simulink model "satcom_4axis_inverse_dinamik"  (R2024b)
settings: Solver=FixedStepDiscrete  StartTime=0.0  StopTime=75.5445  FixedStep=0.0050003  RelTol=1e-3
settings Model: Creator=user  LastModifiedBy=user
settings DataIOCC: ExternalInput=in_qdot_az, in_qddot_az, in_zero, in_zero, in_zero, in_zero, in_zero, in_zero  LoadExternalInput=on

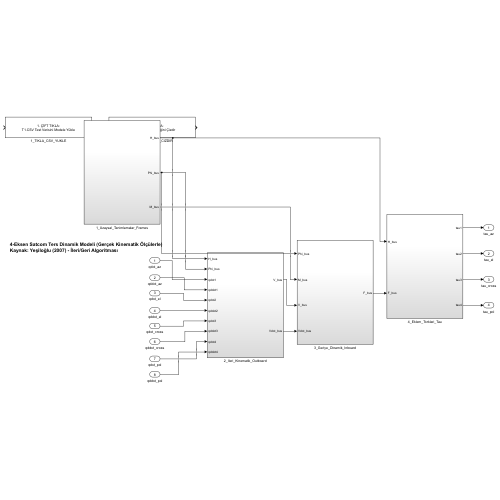
[thumbnail: Simulink's stored preview of the top-level diagram]
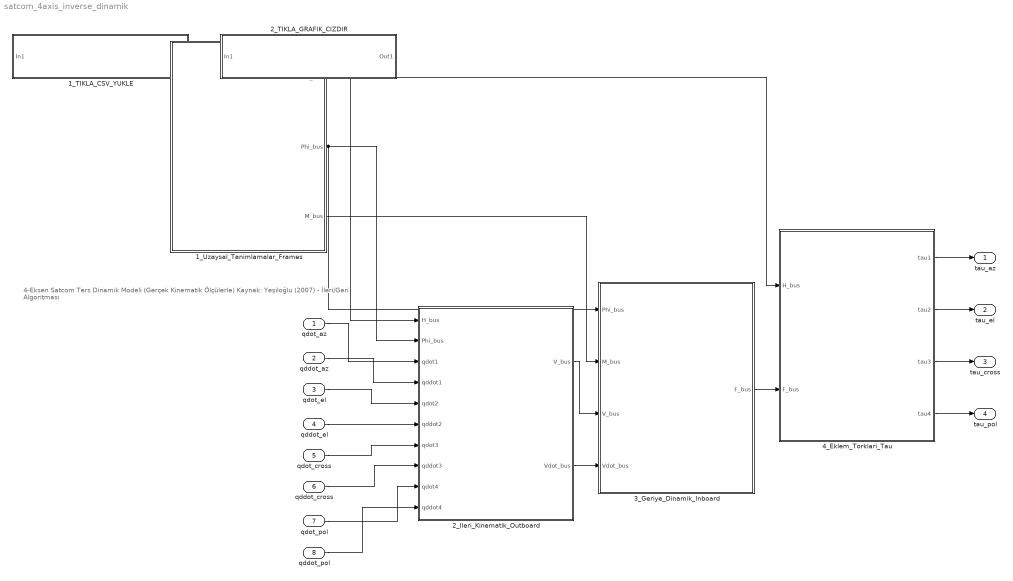
== system satcom_4axis_inverse_dinamik ==
  note: 4-Eksen Satcom Ters Dinamik Modeli (Gerçek Kinematik Ölçülerle)
      | Kaynak: Yeşiloğlu (2007) - İleri/Geri Algoritması
  qdot_az : Inport
  qddot_az : Inport  Port=2
  qdot_el : Inport  Port=3
  qddot_el : Inport  Port=4
  qdot_cross : Inport  Port=5
  qddot_cross : Inport  Port=6
  qdot_pol : Inport  Port=7
  qddot_pol : Inport  Port=8
  1_TIKLA_CSV_YUKLE : Subsystem
      settings: OpenFcn=try, [f,p]=uigetfile({'*.csv;*.xlsx'}); if f~=0, ham_veri = importdata(fullfile(p,f)); if isstruct(ham_veri), mat = ham_veri.data; else, mat = ham_veri; end, t = mat(:,2); t=t(:); v = mat(:,5); v=v(:); a = mat(:,7); a=a(:); akim = mat(:,9); akim=akim(:); tau_real = akim * 1.41; tau_real=tau_real(:); z = zeros(size(t)); dt_array = diff(t); dt_array(dt_array==0)=1e-6; dt_mean = mean(dt_array); assignin('base','in_qdot_az',timeseries(v,t)); assignin('base','in_qddot_az',timeseries(a,t)); assignin('base','in_zero',timeseries(z,t)); assignin('base','csv_zaman',t); assignin('base','csv_tork',tau_real); set_param(bdroot,'SolverType','Fixed-step'); set_param(bdroot,'Solver','FixedStepDiscrete'); set_param(bdroot,'FixedStep',num2str(dt_mean)); set_param(bdroot,'LoadExternalInput','on'); set_param(bdroot,'ExternalInput','in_qdot_az, in_qddot_az, in_zero, in_zero, in_zero, in_zero, in_zero, in_zero'); set_param(bdroot,'StopTime',num2str(t(end))); msgbox('T1.csv verileri yüklendi! Filtreler ve sınırlandırmalar kaldırıldı.', 'BAŞARILI'); end, catch ME, errordlg(sprintf('HATA:\\n%s', ME.message), 'Sistem Hatası'); end
      mask Display: disp('1. ÇİFT TIKLA:\nT1.CSV Test Verisini Modele Yükle');
  1_Uzaysal_Tanimlamalar_Frames : Subsystem
  2_Ileri_Kinematik_Outboard : Subsystem
  2_TIKLA_GRAFIK_CIZDIR : Subsystem
      settings: OpenFcn=try, simOut = evalin('base', 'out'); tau_raw = double(simOut.yout{1}.Values.Data(:)); t_sim = double(simOut.yout{1}.Values.Time(:)); [t_u, idx] = unique(t_sim); tau_u = tau_raw(idx); zaman = evalin('base', 'csv_zaman'); zaman = zaman(:); tau_real = evalin('base', 'csv_tork'); tau_real = tau_real(:); tau_model = interp1(t_u, tau_u, zaman, 'linear', 'extrap'); tau_model = tau_model(:); figure('Name', 'Dinamik Model vs Gerçek Test', 'NumberTitle', 'off'); plot(zaman, tau_model, 'b', 'LineWidth', 1.5); hold on; plot(zaman, tau_real, 'r--', 'LineWidth', 1.2); title('Azimut Motoru - Tork İhtiyacı (Saf Kinematik Model vs Sürücü)'); xlabel('Zaman (s)'); ylabel('Tork (Nm)'); legend('Model Torku (Gerçek Uzuv Mesafeleri İle)', 'Gerçek Sürücü Torku'); grid on; SonucTablosu = table(zaman, tau_model, tau_real, 'VariableNames', {'Zaman_saniye', 'Model_Uretilen_Tork_Nm', 'Gercek_Sistem_Tork_Referansi'}); writetable(SonucTablosu, 'Model_Tork_Sonuclari.csv'); disp('Doğrulama verileri kaydedildi!'); catch ME, errordlg(sprintf('GRAFİK ÇİZİLEMEDİ!\\n\\nHata:\\n%s', ME.message), 'Sistem Hatası'); end
      mask Display: disp('2. ÇİFT TIKLA:\nSaf Model Tork Grafiğini Çizdir');
  3_Geriye_Dinamik_Inboard : Subsystem
  4_Eklem_Torklari_Tau : Subsystem
  tau_az : Outport
  tau_el : Outport  Port=2
  tau_cross : Outport  Port=3
  tau_pol : Outport  Port=4
  wires:
  qdot_az/1 -> 2_Ileri_Kinematik_Outboard/3(qdot1)
  qddot_az/1 -> 2_Ileri_Kinematik_Outboard/4(qddot1)
  qdot_el/1 -> 2_Ileri_Kinematik_Outboard/5(qdot2)
  qddot_el/1 -> 2_Ileri_Kinematik_Outboard/6(qddot2)
  1_Uzaysal_Tanimlamalar_Frames/1(H_bus) -> 4_Eklem_Torklari_Tau/1(H_bus), 2_Ileri_Kinematik_Outboard/1(H_bus)
  qdot_pol/1 -> 2_Ileri_Kinematik_Outboard/9(qdot4)
  qddot_cross/1 -> 2_Ileri_Kinematik_Outboard/8(qddot3)
  qdot_cross/1 -> 2_Ileri_Kinematik_Outboard/7(qdot3)
  4_Eklem_Torklari_Tau/4(tau4) -> tau_pol/1
  4_Eklem_Torklari_Tau/2(tau2) -> tau_el/1
  1_Uzaysal_Tanimlamalar_Frames/2(Phi_bus) -> 3_Geriye_Dinamik_Inboard/1(Phi_bus), 2_Ileri_Kinematik_Outboard/2(Phi_bus)
  1_Uzaysal_Tanimlamalar_Frames/3(M_bus) -> 3_Geriye_Dinamik_Inboard/2(M_bus)
  qddot_pol/1 -> 2_Ileri_Kinematik_Outboard/10(qddot4)
  2_Ileri_Kinematik_Outboard/1(V_bus) -> 3_Geriye_Dinamik_Inboard/3(V_bus)
  2_Ileri_Kinematik_Outboard/2(Vdot_bus) -> 3_Geriye_Dinamik_Inboard/4(Vdot_bus)
  3_Geriye_Dinamik_Inboard/1(F_bus) -> 4_Eklem_Torklari_Tau/2(F_bus)
  4_Eklem_Torklari_Tau/3(tau3) -> tau_cross/1
  4_Eklem_Torklari_Tau/1(tau1) -> tau_az/1

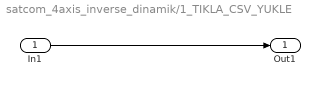
== system satcom_4axis_inverse_dinamik/1_TIKLA_CSV_YUKLE ==
  In1 : Inport
  Out1 : Outport
  wires:
  In1/1 -> Out1/1

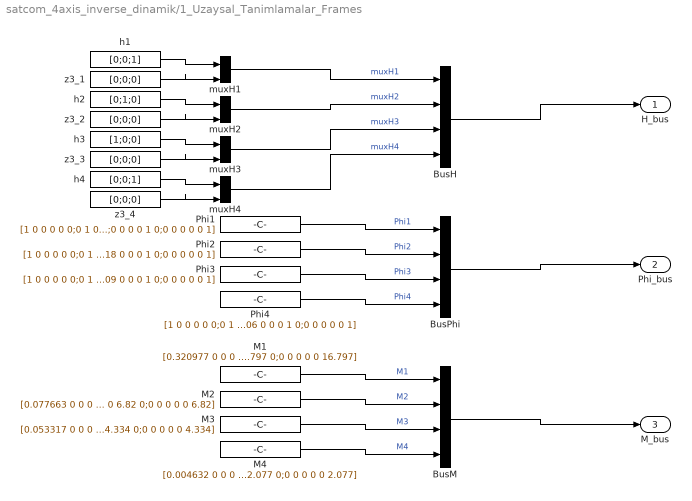
== system satcom_4axis_inverse_dinamik/1_Uzaysal_Tanimlamalar_Frames ==
  BusH : BusCreator  Inputs=4
  BusM : BusCreator  Inputs=4
  BusPhi : BusCreator  Inputs=4
  M1 : Constant  Value=[0.320977 0 0 0 0 0;0 0.320977 0 0 0 0;0 0 0.320977 0 0 0;0 0 0 16.797 0 0;0 0 0 0 16.797 0;0 0 0 0 0 16.797]
  M2 : Constant  Value=[0.077663 0 0 0 0 0;0 0.077663 0 0 0 0;0 0 0.077663 0 0 0;0 0 0 6.82 0 0;0 0 0 0 6.82 0;0 0 0 0 0 6.82]
  M3 : Constant  Value=[0.053317 0 0 0 0 0;0 0.053317 0 0 0 0;0 0 0.053317 0 0 0;0 0 0 4.334 0 0;0 0 0 0 4.334 0;0 0 0 0 0 4.334]
  M4 : Constant  Value=[0.004632 0 0 0 0 0;0 0.004632 0 0 0 0;0 0 0.004632 0 0 0;0 0 0 2.077 0 0;0 0 0 0 2.077 0;0 0 0 0 0 2.077]
  Phi1 : Constant  Value=[1 0 0 0 0 0;0 1 0 0 0 0;0 0 1 0 0 0;0 0 0 1 0 0;0 0 0 0 1 0;0 0 0 0 0 1]
  Phi2 : Constant  Value=[1 0 0 0 0 0;0 1 0 0 0 0;0 0 1 0 0 0;0 0.18 0 1 0 0;-0.18 0 0 0 1 0;0 0 0 0 0 1]
  Phi3 : Constant  Value=[1 0 0 0 0 0;0 1 0 0 0 0;0 0 1 0 0 0;0 0.09 0 1 0 0;-0.09 0 0 0 1 0;0 0 0 0 0 1]
  Phi4 : Constant  Value=[1 0 0 0 0 0;0 1 0 0 0 0;0 0 1 0 0 0;0 0.06 0 1 0 0;-0.06 0 0 0 1 0;0 0 0 0 0 1]
  h1 : Constant  Value=[0;0;1]
  h2 : Constant  Value=[0;1;0]
  h3 : Constant  Value=[1;0;0]
  h4 : Constant  Value=[0;0;1]
  muxH{1..4} (4 alike) : Mux  Inputs=2
  z3_{1..4} (4 alike) : Constant  Value=[0;0;0]
  H_bus : Outport
  Phi_bus : Outport  Port=2
  M_bus : Outport  Port=3
  wires:
  h1/1 -> muxH1/1
  z3_1/1 -> muxH1/2
  muxH1/1 -> BusH/1  "muxH1"
  h2/1 -> muxH2/1
  z3_2/1 -> muxH2/2
  muxH2/1 -> BusH/2  "muxH2"
  h3/1 -> muxH3/1
  z3_3/1 -> muxH3/2
  muxH3/1 -> BusH/3  "muxH3"
  h4/1 -> muxH4/1
  z3_4/1 -> muxH4/2
  muxH4/1 -> BusH/4  "muxH4"
  BusH/1 -> H_bus/1
  Phi1/1 -> BusPhi/1  "Phi1"
  Phi2/1 -> BusPhi/2  "Phi2"
  Phi3/1 -> BusPhi/3  "Phi3"
  Phi4/1 -> BusPhi/4  "Phi4"
  BusPhi/1 -> Phi_bus/1
  M1/1 -> BusM/1  "M1"
  M2/1 -> BusM/2  "M2"
  M3/1 -> BusM/3  "M3"
  M4/1 -> BusM/4  "M4"
  BusM/1 -> M_bus/1

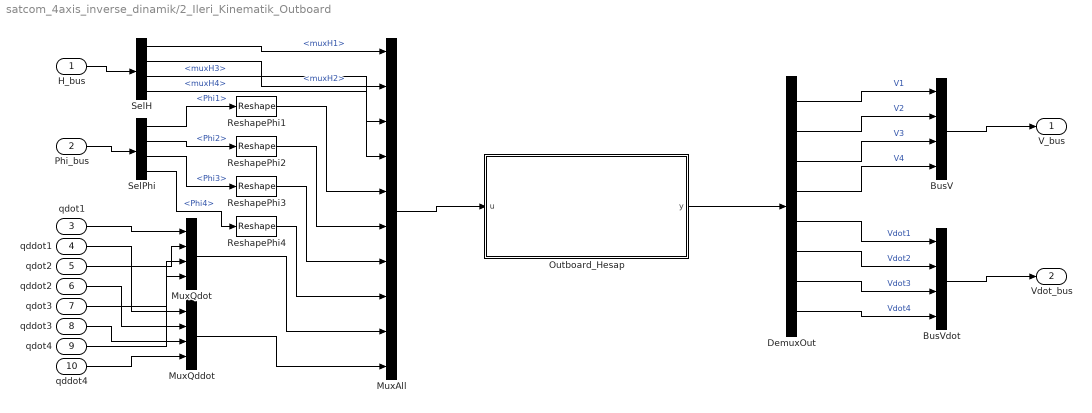
== system satcom_4axis_inverse_dinamik/2_Ileri_Kinematik_Outboard ==
  H_bus : Inport
  Phi_bus : Inport  Port=2
  qdot1 : Inport  Port=3
  qddot1 : Inport  Port=4
  qdot2 : Inport  Port=5
  qddot2 : Inport  Port=6
  qdot3 : Inport  Port=7
  qddot3 : Inport  Port=8
  qdot4 : Inport  Port=9
  qddot4 : Inport  Port=10
  BusV : BusCreator  Inputs=4
  BusVdot : BusCreator  Inputs=4
  DemuxOut : Demux  Outputs=[6 6 6 6 6 6 6 6]
  MuxAll : Mux  Inputs=10
  MuxQddot : Mux
  MuxQdot : Mux
  Outboard_Hesap : MATLAB Function  TreatAsAtomicUnit=on
  ReshapePhi{1..4} (4 alike) : Reshape
  SelH : BusSelector  OutputSignals=muxH1,muxH2,muxH3,muxH4
  SelPhi : BusSelector  OutputSignals=Phi1,Phi2,Phi3,Phi4
  V_bus : Outport
  Vdot_bus : Outport  Port=2
  wires:
  H_bus/1 -> SelH/1
  Phi_bus/1 -> SelPhi/1
  qdot1/1 -> MuxQdot/1
  qddot1/1 -> MuxQddot/1
  qdot2/1 -> MuxQdot/2
  qddot2/1 -> MuxQddot/2
  qdot3/1 -> MuxQdot/3
  qddot3/1 -> MuxQddot/3
  qdot4/1 -> MuxQdot/4
  qddot4/1 -> MuxQddot/4
  SelH/1 -> MuxAll/1  "<muxH1>"
  SelPhi/1 -> ReshapePhi1/1  "<Phi1>"
  ReshapePhi1/1 -> MuxAll/5
  SelH/2 -> MuxAll/2  "<muxH2>"
  SelPhi/2 -> ReshapePhi2/1  "<Phi2>"
  ReshapePhi2/1 -> MuxAll/6
  SelH/3 -> MuxAll/3  "<muxH3>"
  SelPhi/3 -> ReshapePhi3/1  "<Phi3>"
  ReshapePhi3/1 -> MuxAll/7
  SelH/4 -> MuxAll/4  "<muxH4>"
  SelPhi/4 -> ReshapePhi4/1  "<Phi4>"
  ReshapePhi4/1 -> MuxAll/8
  MuxQdot/1 -> MuxAll/9
  MuxQddot/1 -> MuxAll/10
  MuxAll/1 -> Outboard_Hesap/1(u)
  Outboard_Hesap/1(y) -> DemuxOut/1
  DemuxOut/1 -> BusV/1  "V1"
  DemuxOut/5 -> BusVdot/1  "Vdot1"
  DemuxOut/2 -> BusV/2  "V2"
  DemuxOut/6 -> BusVdot/2  "Vdot2"
  DemuxOut/3 -> BusV/3  "V3"
  DemuxOut/7 -> BusVdot/3  "Vdot3"
  DemuxOut/4 -> BusV/4  "V4"
  DemuxOut/8 -> BusVdot/4  "Vdot4"
  BusV/1 -> V_bus/1
  BusVdot/1 -> Vdot_bus/1

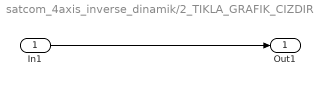
== system satcom_4axis_inverse_dinamik/2_TIKLA_GRAFIK_CIZDIR ==
  In1 : Inport
  Out1 : Outport
  wires:
  In1/1 -> Out1/1

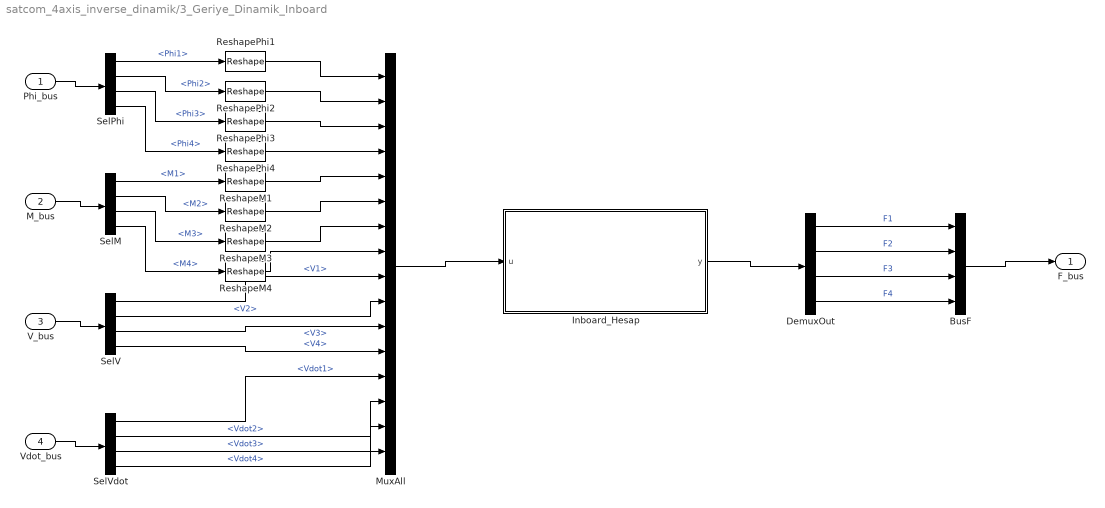
== system satcom_4axis_inverse_dinamik/3_Geriye_Dinamik_Inboard ==
  Phi_bus : Inport
  M_bus : Inport  Port=2
  V_bus : Inport  Port=3
  Vdot_bus : Inport  Port=4
  BusF : BusCreator  Inputs=4
  DemuxOut : Demux  Outputs=[6 6 6 6]
  Inboard_Hesap : MATLAB Function  TreatAsAtomicUnit=on
  MuxAll : Mux  Inputs=16
  ReshapeM{1..4} (4 alike) : Reshape
  ReshapePhi{1..4} (4 alike) : Reshape
  SelM : BusSelector  OutputSignals=M1,M2,M3,M4
  SelPhi : BusSelector  OutputSignals=Phi1,Phi2,Phi3,Phi4
  SelV : BusSelector  OutputSignals=V1,V2,V3,V4
  SelVdot : BusSelector  OutputSignals=Vdot1,Vdot2,Vdot3,Vdot4
  F_bus : Outport
  wires:
  Phi_bus/1 -> SelPhi/1
  M_bus/1 -> SelM/1
  V_bus/1 -> SelV/1
  Vdot_bus/1 -> SelVdot/1
  SelPhi/1 -> ReshapePhi1/1  "<Phi1>"
  ReshapePhi1/1 -> MuxAll/1
  SelM/1 -> ReshapeM1/1  "<M1>"
  ReshapeM1/1 -> MuxAll/5
  SelV/1 -> MuxAll/9  "<V1>"
  SelVdot/1 -> MuxAll/13  "<Vdot1>"
  SelPhi/2 -> ReshapePhi2/1  "<Phi2>"
  ReshapePhi2/1 -> MuxAll/2
  SelM/2 -> ReshapeM2/1  "<M2>"
  ReshapeM2/1 -> MuxAll/6
  SelV/2 -> MuxAll/10  "<V2>"
  SelVdot/2 -> MuxAll/14  "<Vdot2>"
  SelPhi/3 -> ReshapePhi3/1  "<Phi3>"
  ReshapePhi3/1 -> MuxAll/3
  SelM/3 -> ReshapeM3/1  "<M3>"
  ReshapeM3/1 -> MuxAll/7
  SelV/3 -> MuxAll/11  "<V3>"
  SelVdot/3 -> MuxAll/15  "<Vdot3>"
  SelPhi/4 -> ReshapePhi4/1  "<Phi4>"
  ReshapePhi4/1 -> MuxAll/4
  SelM/4 -> ReshapeM4/1  "<M4>"
  ReshapeM4/1 -> MuxAll/8
  SelV/4 -> MuxAll/12  "<V4>"
  SelVdot/4 -> MuxAll/16  "<Vdot4>"
  MuxAll/1 -> Inboard_Hesap/1(u)
  Inboard_Hesap/1(y) -> DemuxOut/1
  DemuxOut/1 -> BusF/1  "F1"
  DemuxOut/2 -> BusF/2  "F2"
  DemuxOut/3 -> BusF/3  "F3"
  DemuxOut/4 -> BusF/4  "F4"
  BusF/1 -> F_bus/1

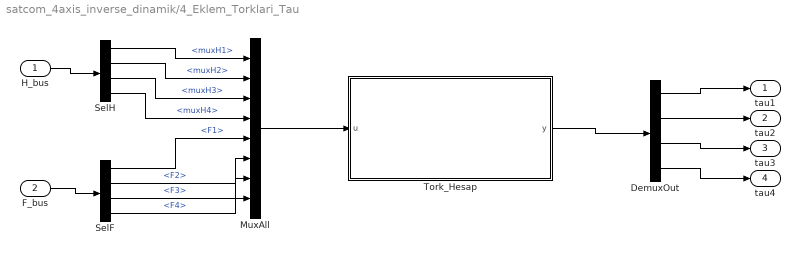
== system satcom_4axis_inverse_dinamik/4_Eklem_Torklari_Tau ==
  H_bus : Inport
  F_bus : Inport  Port=2
  DemuxOut : Demux  Outputs=[1 1 1 1]
  MuxAll : Mux  Inputs=8
  SelF : BusSelector  OutputSignals=F1,F2,F3,F4
  SelH : BusSelector  OutputSignals=muxH1,muxH2,muxH3,muxH4
  Tork_Hesap : MATLAB Function  TreatAsAtomicUnit=on
  tau1 : Outport
  tau2 : Outport  Port=2
  tau3 : Outport  Port=3
  tau4 : Outport  Port=4
  wires:
  H_bus/1 -> SelH/1
  F_bus/1 -> SelF/1
  SelH/1 -> MuxAll/1  "<muxH1>"
  SelF/1 -> MuxAll/5  "<F1>"
  SelH/2 -> MuxAll/2  "<muxH2>"
  SelF/2 -> MuxAll/6  "<F2>"
  SelH/3 -> MuxAll/3  "<muxH3>"
  SelF/3 -> MuxAll/7  "<F3>"
  SelH/4 -> MuxAll/4  "<muxH4>"
  SelF/4 -> MuxAll/8  "<F4>"
  MuxAll/1 -> Tork_Hesap/1(u)
  Tork_Hesap/1(y) -> DemuxOut/1
  DemuxOut/1 -> tau1/1
  DemuxOut/2 -> tau2/1
  DemuxOut/3 -> tau3/1
  DemuxOut/4 -> tau4/1

== matlab function satcom_4axis_inverse_dinamik/2_Ileri_Kinematik_Outboard/Outboard_Hesap ==
  data: u input; y output
function y = fcn(u)
% =========================================================================
% OUTBOARD (ILERI YONLU KINEMATIK) HESAPLAMA BLOGU
% Kaynak: Yesiloglu (2007) - Newton-Euler Ters Dinamik Algoritmasi
% Aciklama: Bu fonksiyonda, kaideden (base) uc is elemanina (end-effector) 
% dogru uzaysal hiz (V) ve uzaysal ivme (Vdot) yayilimini hesapliyorum.
% =========================================================================

H = cell(4,1); Phi = cell(4,1); idx = 1;

% 1. Sinyal Ayiklama: Giris vektorunden H ve Phi matrislerini cekiyoruz
% H: Donme Eksen Vektorleri (Hareket Alt-uzayi matrisleri, 6x1)
for k=1:4, H{k} = u(idx:idx+5); idx = idx + 6; end

% Phi: Uzaysal Donusum (Transfer) Matrisleri (Paralel eksen tasimasi icin, 6x6)
for k=1:4, Phi{k} = reshape(u(idx:idx+35), 6, 6); idx = idx + 36; end

% qdot (Eklem Hizlari) ve qddot (Eklem Ivmeleri)
qdot = u(idx:idx+3); idx = idx + 4; qddot = u(idx:idx+3);

% 2. Baslangic Kosullari: Kaide (Base) sabit oldugu icin hiz ve ivme sifirdir
Vprev = zeros(6,1); Vdotprev = zeros(6,1); V = cell(4,1); Vd = cell(4,1);

% 3. Ileriye Dogru Ozyineleme (Outboard Recursion: 1. eksenden 4. eksene)
for k=1:4
  Vk  = Phi{k}*Vprev + H{k}*qdot(k);
  Vdk = Phi{k}*Vdotprev + H{k}*qddot(k) + crm(Vk)*(H{k}*qdot(k));
  V{k}=Vk; Vd{k}=Vdk; Vprev=Vk; Vdotprev=Vdk;
end

% 4. Cikis Sinyallerini Birlestirme
y = zeros(48,1); idx = 1;
for k=1:4, y(idx:idx+5) = V{k}; idx = idx + 6; end % Uzaysal Hizlar (V1..V4)
for k=1:4, y(idx:idx+5) = Vd{k}; idx = idx + 6; end % Uzaysal Ivmeler (Vdot1..Vdot4)
end

% =========================================================================
% YARDIMCI FONKSIYONLAR
% =========================================================================
function X=crm(V), w=V(1:3); v=V(4:6); X=[skew(w) zeros(3,3); skew(v) skew(w)]; end
function S=skew(a), S=[0 -a(3) a(2); a(3) 0 -a(1); -a(2) a(1) 0]; end

== matlab function satcom_4axis_inverse_dinamik/4_Eklem_Torklari_Tau/Tork_Hesap ==
  data: u input; y output
function y = fcn(u)
H = cell(4,1); F = cell(4,1); idx = 1;
for k=1:4, H{k} = u(idx:idx+5); idx = idx + 6; end
for k=1:4, F{k} = u(idx:idx+5); idx = idx + 6; end
y = zeros(4,1);
for k=1:4
  y(k) = H{k}' * F{k}; 
end
end

== matlab function satcom_4axis_inverse_dinamik/3_Geriye_Dinamik_Inboard/Inboard_Hesap ==
  data: u input; y output
function y = fcn(u)
% =========================================================================
% INBOARD (GERIYE DOGRU DINAMIK) HESAPLAMA BLOGU
% Kaynak: Yesiloglu (2007) - Newton-Euler Ters Dinamik Algoritmasi
% Aciklama: Bu fonksiyonda, en uctaki is elemanindan kaideye dogru 
% geriye isleyerek uzaysal kuvvetlerin yayilimini hesapliyorum.
% =========================================================================

Phi = cell(4,1); I_mat = cell(4,1); V = cell(4,1); Vd = cell(4,1); idx = 1;

% 1. Sinyal Ayiklama: Ileri kinematikten gelen matrisleri ayikliyorum
% Phi: Uzaysal Donusum matrisleri (6x6)
for k=1:4, Phi{k} = reshape(u(idx:idx+35), 6, 6); idx = idx + 36; end

% I_mat: Uzaysal Eylemsizlik matrisleri (6x6)
for k=1:4, I_mat{k} = reshape(u(idx:idx+35), 6, 6); idx = idx + 36; end

% V ve Vd: Uzaysal Hiz ve Uzaysal Ivmeler
for k=1:4, V{k} = u(idx:idx+5); idx = idx + 6; end
for k=1:4, Vd{k} = u(idx:idx+5); idx = idx + 6; end

% 2. Baslangic Kosullari: En uctaki uzva disaridan etki eden yuk yoktur
F=cell(4,1); Fchild=zeros(6,1);

% 3. Geriye Dogru Ozyineleme (Inboard Recursion: 4. eksenden 1. eksene)
for k=4:-1:1
  % --- Newton-Euler Dinamik Denge Denklemi ---
  % Fk: Kendi eylemsizlik kuvvetim + Coriolis/Merkezkac + Alt uzuvdan gelen yuk
  Fk = I_mat{k}*Vd{k} + crf(V{k})*(I_mat{k}*V{k}) + Fchild;
  F{k}=Fk;
  
  % Bu kuvveti donusum matrisinin transpozu ile bir onceki (ebeveyn) uzva tasiyorum
  if k>1, Fchild = Phi{k}' * Fk; end
end

% 4. Cikis Sinyallerini Birlestirme: F1..F4 uzaysal kuvvetlerini disari aktariyorum
y = zeros(24,1); idx = 1;
for k=1:4, y(idx:idx+5) = F{k}; idx = idx + 6; end
end

% =========================================================================
% YARDIMCI FONKSIYONLAR
% =========================================================================
function X=crf(V), X=-crm(V)'; end
function X=crm(V), w=V(1:3); v=V(4:6); X=[skew(w) zeros(3,3); skew(v) skew(w)]; end
function S=skew(a), S=[0 -a(3) a(2); a(3) 0 -a(1); -a(2) a(1) 0]; end
